simulink model "MPPT_PnO"  (R2025b)
settings: Solver=ode3  StartTime=0.0  StopTime=2  FixedStep=1e-5  RelTol=1e-3
libraries: spsSeriesRLCBranchLib x4, spsGroundLib x2, eeGeneralControl x2, spsVoltageMeasurementLib x2, spsCurrentMeasurementLib x1, spsDiodeLib x1, spsMosfetLib x1, spsPVArrayLib x1, spsPWMGeneratorDCDCLib x1, spspowerguiLib x1
settings Model: Creator=hp  LastModifiedBy=hp

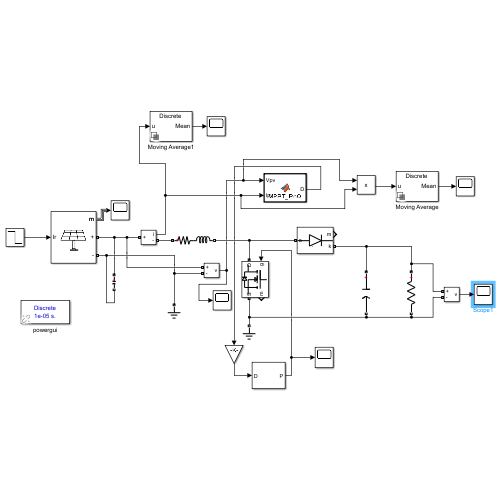
[thumbnail: Simulink's stored preview of the top-level diagram]
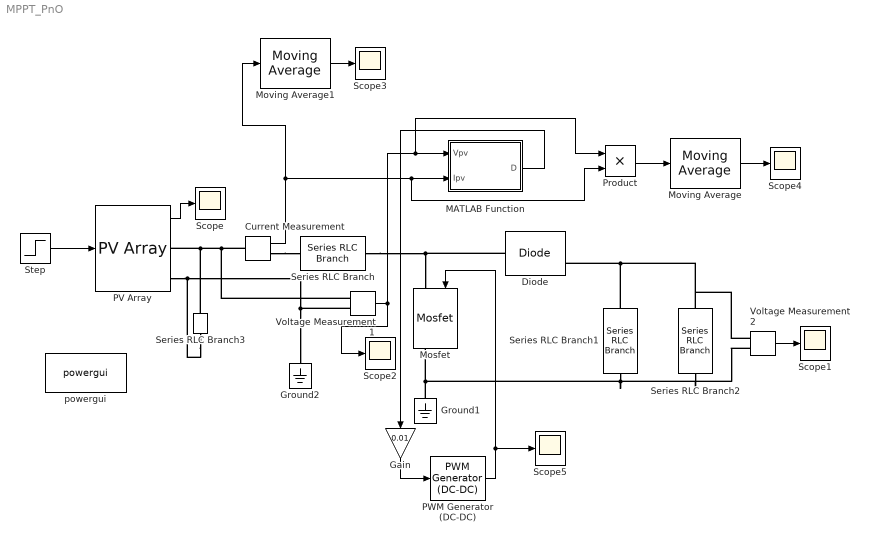
== system MPPT_PnO ==
  Current Measurement : spsCurrentMeasurementLib/Current Measurement  PhasorSimulation=off  OutputType=Complex  PSBequivalent=0
  Diode : spsDiodeLib/Diode  Ron=0.01  Lon=0  Vf=0.8  IC=0  UseSnubber=0  Rs=inf  Cs=0  Measurements=on
  Gain : Gain  Gain=0.01
  Ground1 : spsGroundLib/Ground  LConnTagsString=a
  Ground2 : spsGroundLib/Ground  LConnTagsString=a
  MATLAB Function : MATLAB Function  TreatAsAtomicUnit=on
  Mosfet : spsMosfetLib/Mosfet  Ron=0.01  Lon=0  Rd=0.01  Vfd=0  IC=0  Rs=1e5  Cs=inf  Measurements=on
  Moving Average : eeGeneralControl/Moving Average  VariantControl=Variant1  LabelModeActiveChoice=Discrete  f=10000  x0=0  BufferSize=8192  Ts=1e-5
      settings: LibrarySourceBlock=ee_sl_lib/General Control/Moving Average
  Moving Average1 : eeGeneralControl/Moving Average  VariantControl=Variant1  LabelModeActiveChoice=Discrete  f=10000  x0=0  BufferSize=8192  Ts=1e-5
      settings: LibrarySourceBlock=ee_sl_lib/General Control/Moving Average
  PV Array : spsPVArrayLib/PV Array  Npar=1  Nser=1  PlotType=array @ 25 deg.C & specified irradiances  S_vec="[ 1000  ]"  Temp_C_vec="[ 45 25  ]"  ModuleName=SunPower SPR-305E-WHT-D  PlotWhenSelected=off  Pm=305.226  Ncell=96  Voc=64.2  Isc=5.96  Vm=54.7  Im=5.58  beta_Voc_pc=-0.2727  alpha_Isc_pc=0.061745  beta_Voc=-0.17507  alpha_Isc=0.00368  IL=5.9657  I0=6.3076e-12  nI=0.94489  Rsh=393.2054  Rs=0.37428  RobustModel=on  RobustCellTemperature=25  BAL=on  Tc=1e-6  Tfilter=5e-5
  PWM Generator (DC-DC) : spsPWMGeneratorDCDCLib/PWM Generator (DC-DC)  Fsw=10000  Ts=1e-5
  Product : Product
  Scope{,1..5} (6 alike) : Scope
      Scope settings: ActiveDisplayYMinimum=-1  ActiveDisplayYMaximum=1
      Scope1 settings: ActiveDisplayYMinimum=-8.651071455555293  ActiveDisplayYMaximum=77.859643099997655
      Scope2 settings: ActiveDisplayYMinimum=55  ActiveDisplayYMaximum=70  DataLoggingVariableName=ScopeData2
      Scope3 settings: ActiveDisplayYMinimum=0  ActiveDisplayYMaximum=7  DataLoggingDecimation=10  DataLoggingVariableName=ScopeData3
      Scope4 settings: ActiveDisplayYMinimum=60  ActiveDisplayYMaximum=120  DataLoggingVariableName=ScopeData4
      Scope5 settings: ActiveDisplayYMinimum=-0.14124675712626827  ActiveDisplayYMaximum=1.157593714516751  DataLoggingVariableName=ScopeData5
  Series RLC Branch : spsSeriesRLCBranchLib/Series RLC Branch  LConnTagsString=__new0  RConnTagsString=__new0  BranchType=RL  Resistance=0.01  Inductance=1e-3  SetiL0=off  InitialCurrent=0  Capacitance=1e-6  Setx0=off  InitialVoltage=0  Measurements=None
  Series RLC Branch1 : spsSeriesRLCBranchLib/Series RLC Branch  LConnTagsString=__new0  RConnTagsString=__new0  BranchType=C  Resistance=0.01  Inductance=1e-3  SetiL0=off  InitialCurrent=0  Capacitance=1000e-6  Setx0=off  InitialVoltage=0  Measurements=None
  Series RLC Branch2 : spsSeriesRLCBranchLib/Series RLC Branch  LConnTagsString=__new0  RConnTagsString=__new0  BranchType=R  Resistance=50  Inductance=1e-3  SetiL0=off  InitialCurrent=0  Capacitance=1000e-6  Setx0=off  InitialVoltage=0  Measurements=None
  Series RLC Branch3 : spsSeriesRLCBranchLib/Series RLC Branch  LConnTagsString=__new0  RConnTagsString=__new0  BranchType=C  Resistance=0.01  Inductance=1e-3  SetiL0=off  InitialCurrent=0  Capacitance=1000e-6  Setx0=off  InitialVoltage=0  Measurements=None
  Step : Step  Time=0.3  Before=1000  After=600  SampleTime=0
  Voltage Measurement1 : spsVoltageMeasurementLib/Voltage Measurement  PhasorSimulation=off  OutputType=Complex  PSBequivalent=0
  Voltage Measurement2 : spsVoltageMeasurementLib/Voltage Measurement  PhasorSimulation=off  OutputType=Complex  PSBequivalent=0
  powergui : spspowerguiLib/powergui  Priority=1  SimulationMode=Discrete  SampleTime=1e-5  frequency=60  Iterations=50  frequencyindice=0  Pbase=100e6  ErrMax=1e-4  UnitsV=kV  UnitsW=MW  buscounter=0  FunctionMessages=off  echomessages=off  EnableUseOfTLC=off  CurrentSourceSwitches=off  DisableSnubberDevices=off  DisableRonSwitches=off  DisableVfSwitches=off  DisplayEquations=off  AutomaticDiscreteSolvers=off  SolverType=Tustin/Backward Euler (TBE)  Interpol=off  ExternalGateDelay=off  methode=off  Ts=100  x0status=blocks  SPID=on  SwTol=0  HookPort=off  NonlinearTolerance=1e-4  nMaxIteration=100  ContinueOnMaxIteration=off  RestoreLinks=warning  ResistiveCurrentMeasurement=off  Frange=[0:2:500]  Ylog=off  Xlog=on  ShowGrid=off  save=off  variable=ZData  structure=0  ZoomFFT=off  StartTime=0.0  cycles=1  DisplayStyle=1  fundamental=60  FreqAxis=off  MaxFrequency=1000  frequencyindicesteady=1  RmsSteady=1  display=off
  wires:
  PV Array/1 -> Scope/1
  PWM Generator (DC-DC)/1 -> Mosfet/1, Scope5/1
  Voltage Measurement1/1 -> Product/1, MATLAB Function/1(Vpv), Scope2/1
  Step/1 -> PV Array/1
  Voltage Measurement2/1 -> Scope1/1
  MATLAB Function/1(D) -> Gain/1
  Gain/1 -> PWM Generator (DC-DC)/1
  Product/1 -> Moving Average/1
  Moving Average/1 -> Scope4/1
  Current Measurement/1 -> Moving Average1/1, Product/2, MATLAB Function/2(Ipv)
  Moving Average1/1 -> Scope3/1
  connections:
  PV Array/RConn2 -- Ground2/LConn1 -- Voltage Measurement1/LConn2 -- Series RLC Branch3/RConn1
  Series RLC Branch/RConn1 -- Diode/LConn1 -- Mosfet/LConn1
  Ground1/LConn1 -- Voltage Measurement2/LConn2 -- Series RLC Branch2/RConn1 -- Series RLC Branch1/RConn1 -- Mosfet/RConn1
  Series RLC Branch1/LConn1 -- Voltage Measurement2/LConn1 -- Series RLC Branch2/LConn1 -- Diode/RConn1
  Current Measurement/LConn1 -- Voltage Measurement1/LConn1 -- Series RLC Branch3/LConn1 -- PV Array/RConn1
  Current Measurement/RConn1 -- Series RLC Branch/LConn1

== matlab function MPPT_PnO/MATLAB Function ==
  data: Vpv input; D output; Ipv input
function D = MPPT_PnO(Vpv,Ipv)
persistent Vprev Pprev Dprev counter

if isempty(Vprev)
    Vprev = 0;
    Pprev = 0;
    Dprev = 0.5;  % 50% duty cycle
    counter = 0;
end

% Only update every 5000 steps = 0.05s (with 1e-5 sample time)
counter = counter + 1;

if counter >= 5000  % ← CHANGE THIS
    counter = 0;
    
    P = Vpv * Ipv;
    dP = P - Pprev;
    dV = Vpv - Vprev;
    
    step = 0.002;
    
    if dP > 0
        if dV > 0
            D = Dprev + step;
        else
            D = Dprev - step;
        end
    else
        if dV > 0
            D = Dprev - step;
        else
            D = Dprev + step;
        end
    end
    
    % Limit duty cycle
    D = max(0.3, min(0.8, D));
    
    Vprev = Vpv;
    Pprev = P;
    Dprev = D;
else
    D = Dprev;
end
end
